simulink model "q_dbpen_lin"  (Simulink 7.8)
settings: Solver=ode1  StartTime=0.0  StopTime=inf  FixedStep=0.002  RelTol=1e-3
PostLoadFcn:
  | qc_set_target_type(getConfigSet(bdroot, 'QUARC Default Target Configuration'));
values from neighbouring files (symbols this model uses):
  ALPHA_LIM_ENABLE = 1    [setup_ip02_dbpen.m]
  ALPHA_MAX = 20    [setup_ip02_dbpen.m]
  ALPHA_MIN = - ALPHA_MAX    (= -20)    [setup_ip02_dbpen.m]
  K = [ 0 0 0 0 0 0 0 ]    [setup_ip02_dbpen.m]
  K_AMP = 1    [setup_ip02_dbpen.m]
  VMAX_DAC = 10    [setup_ip02_dbpen.m]
  wcf_1 = 2 * pi * 50.0    (= 314.159265359)    [setup_ip02_dbpen.m]
  wcf_2 = 2 * pi * 10    (= 62.8318530718)    [setup_ip02_dbpen.m]
  X_LIM_ENABLE = 1    [setup_ip02_dbpen.m]
  X_MAX = 0.40    (= 0.4)    [setup_ip02_dbpen.m]
  X_MIN = - X_MAX    (= -0.4)    [setup_ip02_dbpen.m]
  zetaf_1 = 0.9    [setup_ip02_dbpen.m]
  zetaf_2 = 0.9    [setup_ip02_dbpen.m]
undefined symbols (not defined in the file or in its folder): HIL, K_EC, K_EP, qc_get_step_size, VMAX_AMP
libraries: quarc_library x9, simulink_extras x5
settings Model: Creator=Mfotoohi  LastModifiedBy=pmartin  SimulationMode=external  ExtModeTrigDuration=20000
settings SolverCC: PositivePriorityOrder=on
settings OptimizationCC: BooleanDataType=off  InitFltsAndDblsToZero=on
settings DebuggingCC: SaveWithParameterizedLinksMsg=none  MultiTaskDSMMsg=warning  MultiTaskCondExecSysMsg=none  FcnCallInpInsideContextMsg=Use local settings  StrictBusMsg=None
settings HardwareCC: TargetHWDeviceType=32-bit Generic
settings RTWCC: SystemTargetFile=quarc_windows.tlc  TemplateMakefile=quarc_default_tmf  Description=QUARC Win32 Target  ProcessScript=quarc_windows_make_rtw_hook  IncludeERTFirstTime=on
settings STFCustomTargetCC: TargetPreCompLibLocation=C:\PROGRA~2\QUARC\lib\2011b\windows\release  SystemTargetFile=quarc_windows.tlc
settings GRTTargetCC: TargetPreCompLibLocation=C:\PROGRA~2\QUARC\lib\2011b\windows\release  ParMdlRefBuildCompliant=off  CompOptLevelCompliant=off  ConcurrentExecutionCompliant=off  MatFileLogging=off  ExtMode=on  ExtModeMexFile=quarc_comm

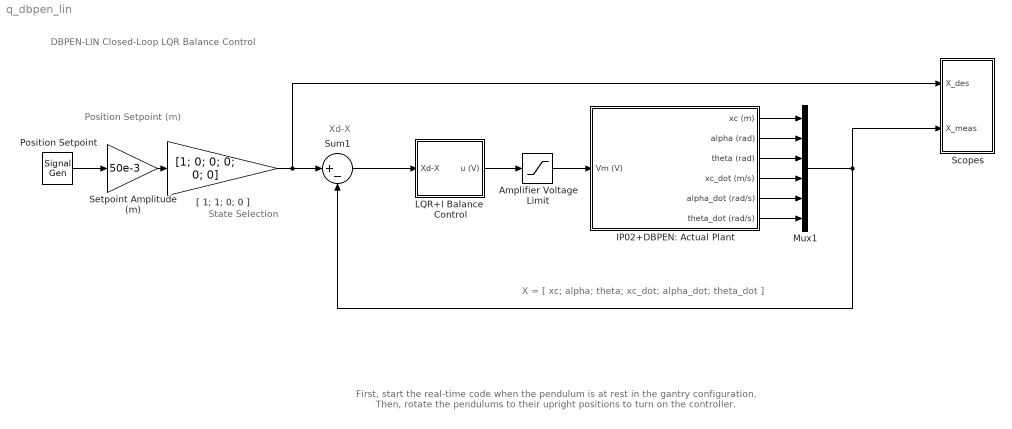
== system q_dbpen_lin ==
  note: DBPEN-LIN Closed-Loop
      | LQR Balance Control
  note: X = [ xc; alpha; theta; xc_dot; alpha_dot; theta_dot ]
  note: Xd-X
  note: State Selection
  note: Position Setpoint (m)
  note: First, start the real-time code when the pendulum is at rest in the gantry configuration.
      | Then, rotate the pendulums to their upright positions to turn on the controller.
  Amplifier Voltage Limit : Saturate  UpperLimit=VMAX_AMP  LowerLimit=- VMAX_AMP
  IP02+DBPEN: Actual Plant : Subsystem
  LQR+I Balance  Control : Subsystem
  Mux1 : Mux  Inputs=6
  Position Setpoint : SignalGenerator  WaveForm=square  Frequency=0.05
  Scopes : Subsystem
  Setpoint Amplitude (m) : Gain  Gain=50e-3  SaturateOnIntegerOverflow=on  OutDataTypeStr=Inherit: Same as input  ParamDataTypeStr=Inherit: Same as input
  Sum1 : Sum  Inputs=|+-  SaturateOnIntegerOverflow=on  InputSameDT=on  OutDataTypeStr=Inherit: Same as first input
  "[ 1; 1; 0; 0 ]" : Gain  Gain=[1; 0; 0; 0; 0; 0]  SaturateOnIntegerOverflow=on  OutDataTypeStr=Inherit: Same as input  ParamDataTypeStr=Inherit: Same as input
  wires:
  Amplifier Voltage Limit/1 -> IP02+DBPEN: Actual Plant/1(Vm (V))
  "[ 1; 1; 0; 0 ]"/1 -> Sum1/1, Scopes/1(X_des)
  Mux1/1 -> Scopes/2(X_meas), Sum1/2
  Position Setpoint/1 -> Setpoint Amplitude (m)/1
  Setpoint Amplitude (m)/1 -> "[ 1; 1; 0; 0 ]"/1
  IP02+DBPEN: Actual Plant/1(xc (m)) -> Mux1/1
  IP02+DBPEN: Actual Plant/2(alpha (rad)) -> Mux1/2
  IP02+DBPEN: Actual Plant/3(theta (rad)) -> Mux1/3
  IP02+DBPEN: Actual Plant/4(xc_dot (m/s)) -> Mux1/4
  IP02+DBPEN: Actual Plant/5(alpha_dot (rad/s)) -> Mux1/5
  IP02+DBPEN: Actual Plant/6(theta_dot (rad/s)) -> Mux1/6
  LQR+I Balance  Control/1(u (V)) -> Amplifier Voltage Limit/1
  Sum1/1 -> LQR+I Balance  Control/1(Xd-X)

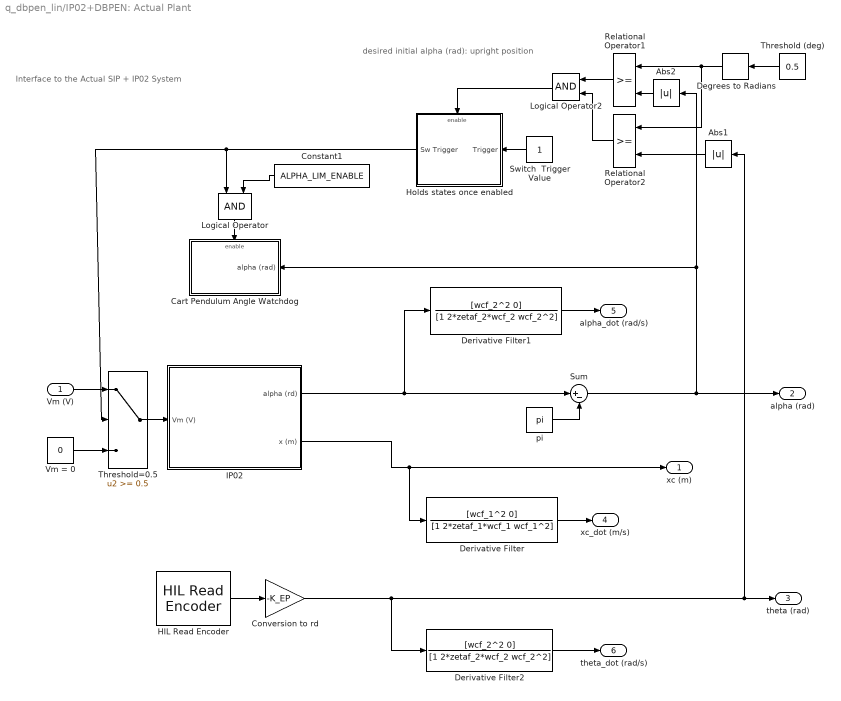
== system q_dbpen_lin/IP02+DBPEN: Actual Plant ==
  note: desired initial alpha (rad):
      | upright position
  note: Interface to the Actual
      | SIP + IP02 System
  Vm (V) : Inport
  Abs1 : Abs  SaturateOnIntegerOverflow=on
  Abs2 : Abs  SaturateOnIntegerOverflow=on
  Cart Pendulum Angle Watchdog : Subsystem  TreatAsAtomicUnit=on
  Constant1 : Constant  Value=ALPHA_LIM_ENABLE  OutDataTypeStr=double
  Conversion to rd : Gain  Gain=-K_EP  SaturateOnIntegerOverflow=on  OutDataTypeStr=Inherit: Same as input  ParamDataTypeStr=Inherit: Same as input
  Degrees to Radians : simulink_extras/Transformations/Degrees to Radians
  Derivative Filter : TransferFcn  Numerator=[wcf_1^2 0]  Denominator=[1 2*zetaf_1*wcf_1 wcf_1^2]
  Derivative Filter1 : TransferFcn  Numerator=[wcf_2^2 0]  Denominator=[1 2*zetaf_2*wcf_2 wcf_2^2]
  Derivative Filter2 : TransferFcn  Numerator=[wcf_2^2 0]  Denominator=[1 2*zetaf_2*wcf_2 wcf_2^2]
  HIL Read Encoder : quarc_library/Data Acquisition/Generic/Immediate I//O/HIL Read Encoder  object_name=HIL-1  channels=2  sample_time=qc_get_step_size  active=on  vector_output=off  data_type_mode=Inherit via back propagation  data_type=double
  Holds states once enabled : Subsystem  TreatAsAtomicUnit=on
  "IP02 " : Subsystem
  Logical Operator : Logic
  Logical Operator2 : Logic
  Relational Operator1 : RelationalOperator  InputSameDT=on
  Relational Operator2 : RelationalOperator  InputSameDT=on
  Sum : Sum  Inputs=|+-  SaturateOnIntegerOverflow=on  InputSameDT=on  OutDataTypeStr=Inherit: Same as first input
  Switch  Trigger Value : Constant
  Threshold (deg) : Constant  Value=0.5
  Threshold=0.5 : Switch  Threshold=0.5  SaturateOnIntegerOverflow=on  InputSameDT=on
  Vm = 0 : Constant  Value=0
  pi : Constant  Value=pi
  xc (m) : Outport  InitialOutput=0
  alpha (rad) : Outport  Port=2  InitialOutput=0
  theta (rad) : Outport  Port=3  InitialOutput=0
  xc_dot (m/s) : Outport  Port=4  InitialOutput=0
  alpha_dot (rad/s) : Outport  Port=5  InitialOutput=0
  theta_dot (rad/s) : Outport  Port=6  InitialOutput=0
  wires:
  Relational Operator2/1 -> Logical Operator2/2
  Threshold (deg)/1 -> Degrees to Radians/1
  Abs1/1 -> Relational Operator2/2
  Abs2/1 -> Relational Operator1/2
  Relational Operator1/1 -> Logical Operator2/1
  Logical Operator2/1 -> Holds states once enabled/Enable
  Derivative Filter2/1 -> theta_dot (rad/s)/1
  Conversion to rd/1 -> Abs1/1, theta (rad)/1, Derivative Filter2/1
  HIL Read Encoder/1 -> Conversion to rd/1
  Constant1/1 -> Logical Operator/2
  Logical Operator/1 -> Cart Pendulum Angle Watchdog/Enable
  Sum/1 -> Abs2/1, Cart Pendulum Angle Watchdog/1(alpha (rad)), alpha (rad)/1
  pi/1 -> Sum/2
  Vm = 0/1 -> Threshold=0.5/3
  Vm (V)/1 -> Threshold=0.5/1
  Holds states once enabled/1(Sw Trigger) -> Logical Operator/1, Threshold=0.5/2
  Threshold=0.5/1 -> "IP02 "/1(Vm (V))
  Switch  Trigger Value/1 -> Holds states once enabled/1(Trigger)
  Degrees to Radians/1 -> Relational Operator2/1, Relational Operator1/1
  Derivative Filter/1 -> xc_dot (m/s)/1
  "IP02 "/1(alpha (rd)) -> Sum/1, Derivative Filter1/1
  Derivative Filter1/1 -> alpha_dot (rad/s)/1
  "IP02 "/2(x (m)) -> Derivative Filter/1, xc (m)/1

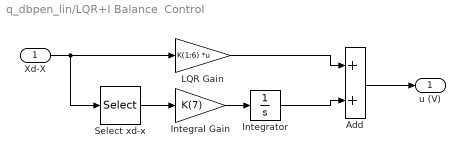
== system q_dbpen_lin/LQR+I Balance  Control ==
  Xd-X : Inport
  Add : Sum
  Integral Gain : Gain  Gain=K(7)
  Integrator : Integrator  LimitOutput=on  UpperSaturationLimit=4  LowerSaturationLimit=-4
  LQR Gain : Gain  Gain=K(1:6)  Multiplication=Matrix(K*u)
  Select xd-x : Selector  InputPortWidth=6  IndexOptions=Index vector (dialog)  Indices=[1]  OutputSizes=1
  u (V) : Outport
  wires:
  Xd-X/1 -> LQR Gain/1, Select xd-x/1
  Integral Gain/1 -> Integrator/1
  LQR Gain/1 -> Add/1
  Integrator/1 -> Add/2
  Add/1 -> u (V)/1
  Select xd-x/1 -> Integral Gain/1

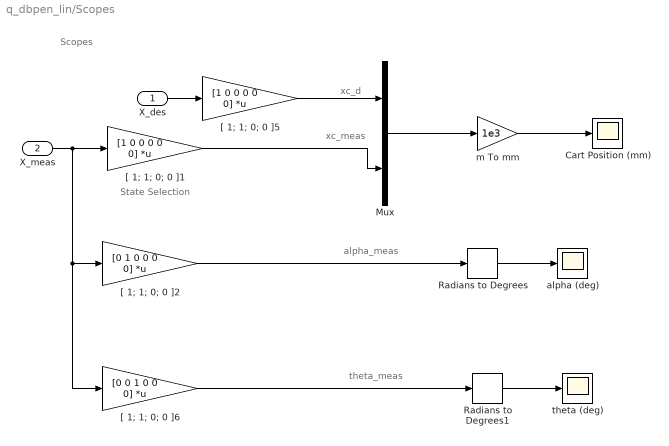
== system q_dbpen_lin/Scopes ==
  note: xc_meas
  note: State Selection
  note: alpha_meas
  note: xc_d
  note: Scopes
  note: theta_meas
  X_des : Inport
  X_meas : Inport  Port=2
  Cart Position (mm) : Scope
      settings: TickLabels=on  TimeRange=20  YMin=-200  YMax=200  SaveName=data_xc  DataFormat=Array  MaxDataPoints=20000
  Mux : Mux  Inputs=2
  Radians to Degrees : simulink_extras/Transformations/Radians to Degrees
  Radians to Degrees1 : simulink_extras/Transformations/Radians to Degrees
  "[ 1; 1; 0; 0 ]1" : Gain  Gain=[1 0 0 0 0 0]  Multiplication=Matrix(K*u)  SaturateOnIntegerOverflow=on  OutDataTypeStr=Inherit: Same as input  ParamDataTypeStr=Inherit: Same as input
  "[ 1; 1; 0; 0 ]2" : Gain  Gain=[0 1 0 0 0 0]  Multiplication=Matrix(K*u)  SaturateOnIntegerOverflow=on  OutDataTypeStr=Inherit: Same as input  ParamDataTypeStr=Inherit: Same as input
  "[ 1; 1; 0; 0 ]5" : Gain  Gain=[1 0 0 0 0 0]  Multiplication=Matrix(K*u)  SaturateOnIntegerOverflow=on  OutDataTypeStr=Inherit: Same as input  ParamDataTypeStr=Inherit: Same as input
  "[ 1; 1; 0; 0 ]6" : Gain  Gain=[0 0 1 0 0 0]  Multiplication=Matrix(K*u)  SaturateOnIntegerOverflow=on  OutDataTypeStr=Inherit: Same as input  ParamDataTypeStr=Inherit: Same as input
  alpha (deg) : Scope
      settings: TickLabels=on  TimeRange=20  YMin=-200  YMax=200  SaveName=data_alpha  DataFormat=Array  MaxDataPoints=20000
  m To mm : Gain  Gain=1e3  SaturateOnIntegerOverflow=on  OutDataTypeStr=Inherit: Same as input  ParamDataTypeStr=Inherit: Same as input
  theta (deg) : Scope
      settings: TickLabels=on  TimeRange=20  YMin=-200  YMax=200  SaveName=data_theta  DataFormat=Array  MaxDataPoints=20000
  wires:
  Mux/1 -> m To mm/1
  m To mm/1 -> Cart Position (mm)/1
  "[ 1; 1; 0; 0 ]1"/1 -> Mux/2
  X_des/1 -> "[ 1; 1; 0; 0 ]5"/1
  X_meas/1 -> "[ 1; 1; 0; 0 ]1"/1, "[ 1; 1; 0; 0 ]2"/1, "[ 1; 1; 0; 0 ]6"/1
  Radians to Degrees/1 -> alpha (deg)/1
  "[ 1; 1; 0; 0 ]5"/1 -> Mux/1
  "[ 1; 1; 0; 0 ]2"/1 -> Radians to Degrees/1
  Radians to Degrees1/1 -> theta (deg)/1
  "[ 1; 1; 0; 0 ]6"/1 -> Radians to Degrees1/1

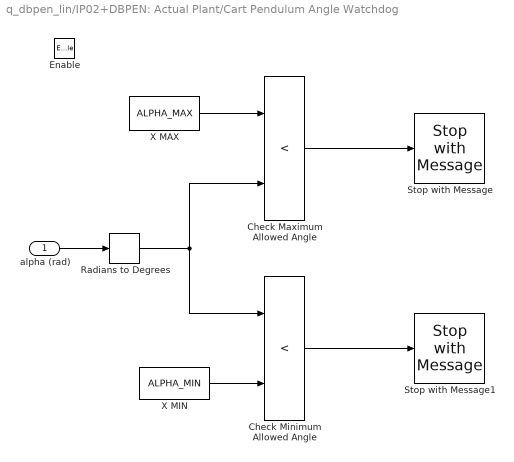
== system q_dbpen_lin/IP02+DBPEN: Actual Plant/Cart Pendulum Angle Watchdog ==
  alpha (rad) : Inport
  Enable : EnablePort
  Check Maximum Allowed Angle : RelationalOperator  Operator=<  InputSameDT=on
  Check Minimum Allowed Angle : RelationalOperator  Operator=<  InputSameDT=on
  Radians to Degrees : simulink_extras/Transformations/Radians to Degrees
  Stop with Message : quarc_library/Sinks/Error Handling/Stop with Message  message_type=Fixed error message  message_icon=Warning  message=Maximum Angle Reached.
  Stop with Message1 : quarc_library/Sinks/Error Handling/Stop with Message  message_type=Fixed error message  message_icon=Warning  message=Minimum Angle Reached.
  X MAX : Constant  Value=ALPHA_MAX
  X MIN : Constant  Value=ALPHA_MIN
  wires:
  Radians to Degrees/1 -> Check Minimum Allowed Angle/1, Check Maximum Allowed Angle/2
  Check Maximum Allowed Angle/1 -> Stop with Message/1
  alpha (rad)/1 -> Radians to Degrees/1
  X MIN/1 -> Check Minimum Allowed Angle/2
  Check Minimum Allowed Angle/1 -> Stop with Message1/1
  X MAX/1 -> Check Maximum Allowed Angle/1

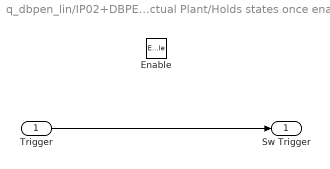
== system q_dbpen_lin/IP02+DBPEN: Actual Plant/Holds states once enabled ==
  Trigger : Inport  OutDataTypeStr=double
  Enable : EnablePort
  Sw Trigger : Outport  OutDataTypeStr=double  InitialOutput=[0]
  wires:
  Trigger/1 -> Sw Trigger/1

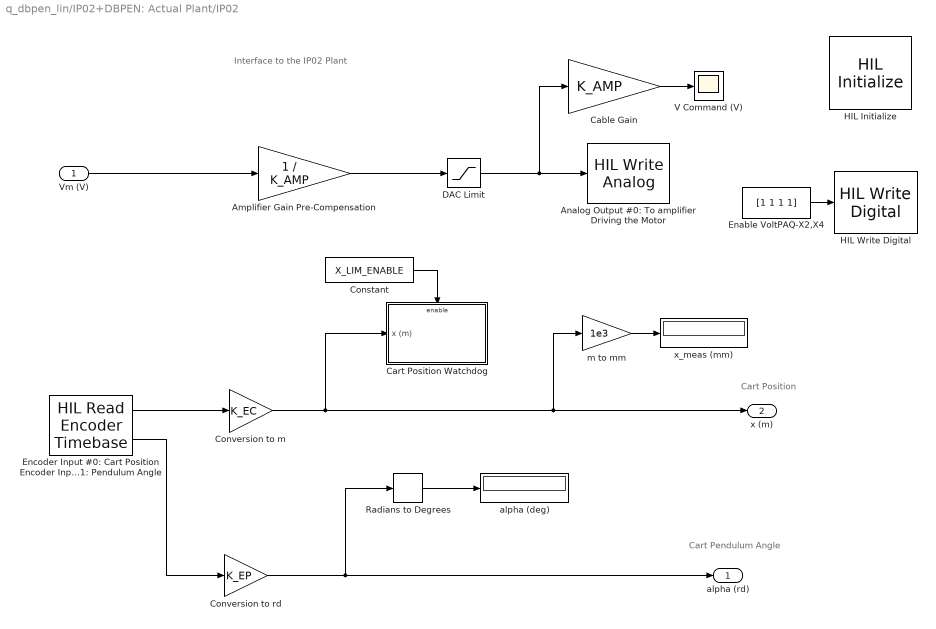
== system q_dbpen_lin/IP02+DBPEN: Actual Plant/IP02  ==
  note: Interface to the IP02 Plant
  note: Cart Position
  note: Cart Pendulum Angle
  Vm (V) : Inport
  Amplifier Gain Pre-Compensation : Gain  Gain=1 / K_AMP  SaturateOnIntegerOverflow=on  OutDataTypeStr=Inherit: Same as input  ParamDataTypeStr=Inherit: Same as input
  Analog Output #0: To amplifier Driving the Motor : quarc_library/Data Acquisition/Generic/Immediate I//O/HIL Write Analog  Tag=unassigned  object_name=HIL-1  channels=0  sample_time=-1  active=on  vector_input=on
  Cable Gain : Gain  Gain=K_AMP  SaturateOnIntegerOverflow=on  OutDataTypeStr=Inherit: Same as input  ParamDataTypeStr=Inherit: Same as input
  Cart Position Watchdog : Subsystem  TreatAsAtomicUnit=on
  Constant : Constant  Value=X_LIM_ENABLE
  Conversion to m : Gain  Gain=K_EC  SaturateOnIntegerOverflow=on  OutDataTypeStr=Inherit: Same as input  ParamDataTypeStr=Inherit: Same as input
  Conversion to rd : Gain  Gain=K_EP  SaturateOnIntegerOverflow=on  OutDataTypeStr=Inherit: Same as input  ParamDataTypeStr=Inherit: Same as input
  DAC Limit : Saturate  UpperLimit=VMAX_DAC  LowerLimit=- VMAX_DAC
  Enable VoltPAQ-X2,X4 : Constant  Value=[1 1 1 1]
  Encoder Input #0: Cart Position Encoder Input #1: Pendulum Angle : quarc_library/Data Acquisition/Generic/Timebases/HIL Read Encoder Timebase  object_name=HIL-1  clock=0  channels=[0:1]  samples_in_buffer=max(ceil(1/qc_get_step_size), 1)  active=on  vector_output=off  data_type_mode=Inherit via back propagation  data_type=double
  HIL Initialize : quarc_library/Data Acquisition/Generic/Configuration/HIL Initialize  object_name=HIL-1  board_type=q8_usb  board_number=0  board_options=update_rate=normal  exclusive=off  active=off  hardware_clocks=[0:2]  clock_modes=[]  initial_clock_frequencies=[]  set_clock_params_at_start=off  set_clock_params_at_switch_in=off  set_clock_frequencies_at_start=off  set_clock_frequencies_at_switch_in=off  analog_input_channels=[0:7]  analog_input_maximums=10  analog_input_minimums=-10  set_analog_input_params_at_start=on  set_analog_input_params_at_switch_in=off  analog_output_channels=[0:7]  analog_output_maximums=10  analog_output_minimums=-10  initial_analog_outputs=[0]  final_analog_outputs=[0]  watchdog_analog_outputs=0  set_analog_output_params_at_start=on  set_analog_output_params_at_switch_in=off  set_analog_outputs_at_start=on  set_analog_outputs_at_switch_in=off  set_analog_outputs_at_terminate=on  set_analog_outputs_at_switch_out=off  set_analog_outputs_on_watchdog=off  digital_input_channels=[]  digital_output_channels=[0:7]  digital_output_configuration=[]  initial_digital_outputs=[0]  final_digital_outputs=[0]  watchdog_digital_outputs=[0]  set_digital_output_params_at_start=off  set_digital_output_params_at_switch_in=off  set_digital_outputs_at_start=on  set_digital_outputs_at_switch_in=off  set_digital_outputs_at_terminate=on  set_digital_outputs_at_switch_out=off  set_digital_outputs_on_watchdog=off  encoder_channels=[0:7]  quadrature=[4]  encoder_filter_frequency=[]  initial_encoder_counts=[0]  set_encoder_params_at_start=on  set_encoder_params_at_switch_in=off  set_encoder_counts_at_start=on  set_encoder_counts_at_switch_in=off  pwm_channels=[0:7]  pwm_modes=0  pwm_frequency=99.532799999999995e6/4095  pwm_configuration=[0]  pwm_alignment=[0]  pwm_polarity=[1]  pwm_leading_deadband=[0]  pwm_trailing_deadband=[0]  initial_pwm_outputs=[0]  final_pwm_outputs=[0]  watchdog_pwm_outputs=[0]  set_pwm_params_at_start=on  set_pwm_params_at_switch_in=off  set_pwm_outputs_at_start=on  set_pwm_outputs_at_switch_in=off  set_pwm_outputs_at_terminate=on  set_pwm_outputs_at_switch_out=off  set_pwm_outputs_on_watchdog=off  other_output_channels=[]  initial_other_outputs=[]  final_other_outputs=[]  watchdog_other_outputs=[]  set_other_outputs_at_start=off  set_other_outputs_at_switch_in=off  set_other_outputs_at_terminate=off  set_other_outputs_at_switch_out=off  set_other_outputs_on_watchdog=off
  HIL Write Digital : quarc_library/Data Acquisition/Generic/Immediate I//O/HIL Write Digital  object_name=HIL-1  channels=[0:3]  sample_time=-1  active=off  vector_input=on
  Radians to Degrees : simulink_extras/Transformations/Radians to Degrees
  V Command (V) : Scope
      settings: TickLabels=on  TimeRange=20  YMin=-10  YMax=10  SaveName=data_Vm  DataFormat=Array  MaxDataPoints=20000
  alpha (deg) : Display
  m to mm : Gain  Gain=1e3  SaturateOnIntegerOverflow=on  OutDataTypeStr=Inherit: Same as input  ParamDataTypeStr=Inherit: Same as input
  x_meas (mm) : Display
      settings: Decimation=100
  alpha (rd) : Outport  InitialOutput=0
  x (m) : Outport  Port=2  InitialOutput=0
  wires:
  Enable VoltPAQ-X2,X4/1 -> HIL Write Digital/1
  Constant/1 -> Cart Position Watchdog/Enable
  Cable Gain/1 -> V Command (V)/1
  Vm (V)/1 -> Amplifier Gain Pre-Compensation/1
  DAC Limit/1 -> Cable Gain/1, Analog Output #0: To amplifier Driving the Motor/1
  Conversion to rd/1 -> alpha (rd)/1, Radians to Degrees/1
  Radians to Degrees/1 -> alpha (deg)/1
  Encoder Input #0: Cart Position Encoder Input #1: Pendulum Angle/2 -> Conversion to rd/1
  m to mm/1 -> x_meas (mm)/1
  Amplifier Gain Pre-Compensation/1 -> DAC Limit/1
  Conversion to m/1 -> m to mm/1, x (m)/1, Cart Position Watchdog/1(x (m))
  Encoder Input #0: Cart Position Encoder Input #1: Pendulum Angle/1 -> Conversion to m/1

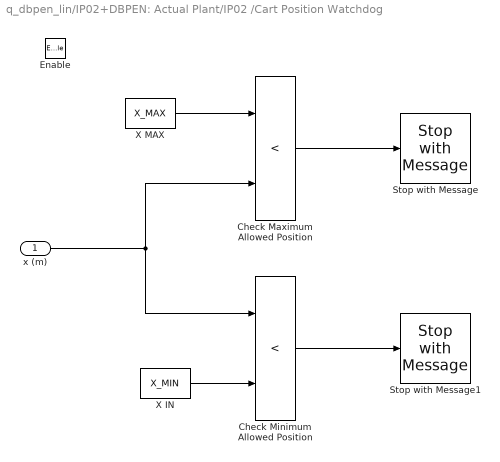
== system q_dbpen_lin/IP02+DBPEN: Actual Plant/IP02 /Cart Position Watchdog ==
  x (m) : Inport
  Enable : EnablePort
  Check Maximum Allowed Position : RelationalOperator  Operator=<  InputSameDT=on
  Check Minimum Allowed Position : RelationalOperator  Operator=<  InputSameDT=on
  Stop with Message : quarc_library/Sinks/Error Handling/Stop with Message  message_type=Fixed error message  message_icon=Warning  message=Maximum Cart Limit Reached.
  Stop with Message1 : quarc_library/Sinks/Error Handling/Stop with Message  message_type=Fixed error message  message_icon=Warning  message=Minimum Cart Limit Reached.
  X IN : Constant  Value=X_MIN
  X MAX : Constant  Value=X_MAX
  wires:
  X MAX/1 -> Check Maximum Allowed Position/1
  Check Minimum Allowed Position/1 -> Stop with Message1/1
  X IN/1 -> Check Minimum Allowed Position/2
  x (m)/1 -> Check Maximum Allowed Position/2, Check Minimum Allowed Position/1
  Check Maximum Allowed Position/1 -> Stop with Message/1
